simulink model "nichtlinearesModell_Kalman"  (R2016b)
settings: Solver=VariableStepAuto  StartTime=0.0  StopTime=30  RelTol=1e-3
values from neighbouring files (symbols this model uses):
  Ak = [A1                      E*C_s ... (first row only)    [StartSim.m]
  B1 = [0 b2 0 b4]'    [RiccatiBerechnung_Anlage.m]    (also in RiccatiBerechnunguPlot_Simulation.m; StartSim.m)
  Bk = [B1; zeros(1,size(B1,2))]    [StartSim.m]
  Ck = [C1 zeros(size(C1,1),1)]    [StartSim.m]
  K1 = 1    [RiccatiBerechnung_Anlage.m]    (also in RiccatiBerechnunguPlot_Simulation.m; StartSim.m)
  K2 = 1    [RiccatiBerechnung_Anlage.m]    (also in RiccatiBerechnunguPlot_Simulation.m; StartSim.m)
  Kk = P * Ck' / R    [StartSim.m]
  L_0 = 0.5    [RiccatiBerechnunguPlot_Simulation.m]    (also in StartSim.m)
  phi_0 = 0    [RiccatiBerechnunguPlot_Simulation.m]    (also in StartSim.m)
  r1 = 0.0191    [LQG.m]    (also in RiccatiBerechnung_Anlage.m = 0.046; RiccatiBerechnunguPlot_Simulation.m = 0.046; StartSim.m = 0.046)
  r2 = 0.015915    [LQG.m]    (also in RiccatiBerechnung_Anlage.m = 0.021975; RiccatiBerechnunguPlot_Simulation.m = 0.021975; StartSim.m = 0.025)
  T1 = 0.1    [LQG.m]    (also in RiccatiBerechnung_Anlage.m = 0.03032; RiccatiBerechnunguPlot_Simulation.m = 0.03032; StartSim.m = 0.03032)
  T2 = 0.1    [LQG.m]    (also in RiccatiBerechnung_Anlage.m = 0.0247; RiccatiBerechnunguPlot_Simulation.m = 0.0247; StartSim.m = 0.03032)
  ue1 = 6    [RiccatiBerechnung_Anlage.m]    (also in RiccatiBerechnunguPlot_Simulation.m; StartSim.m)
  ue2 = 3    [RiccatiBerechnung_Anlage.m]    (also in RiccatiBerechnunguPlot_Simulation.m; StartSim.m)
  x_0 = 2.54    [RiccatiBerechnunguPlot_Simulation.m]    (also in StartSim.m = 1.3)
undefined symbols (not defined in the file or in its folder): K
libraries: simulink_extras x3, simulink x2
settings Model: Creator=Patrick  LastModifiedBy=Patrick

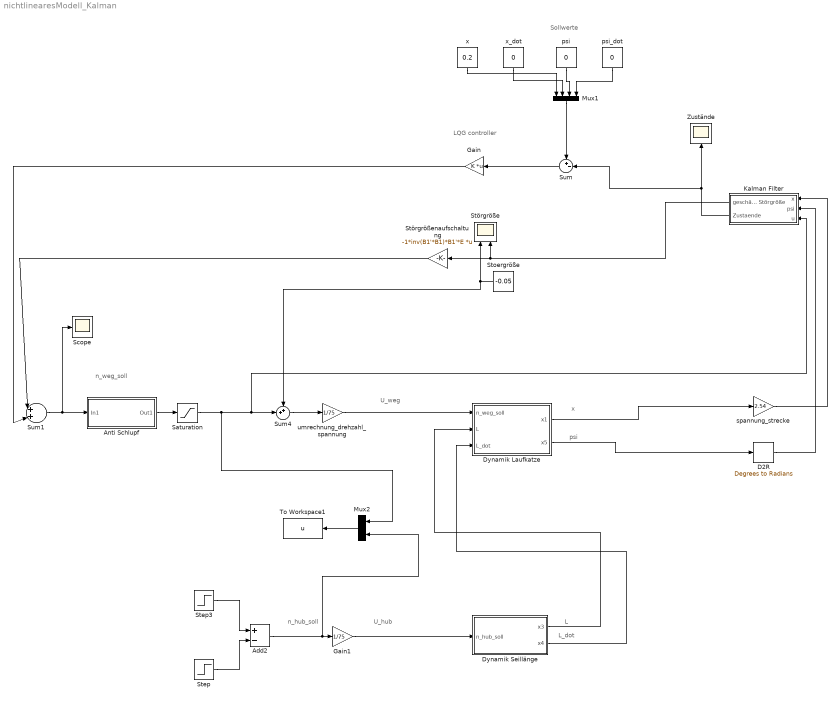
== system nichtlinearesModell_Kalman ==
  note: n_hub_soll
  note: U_hub
  note: L
  note: L_dot
  note: x
  note: psi
  note: LQG controller
  note: U_weg
  note: n_weg_soll
  note: Sollwerte
  Add2 : Sum  Inputs=+-
  Anti Schlupf : Subsystem
  D2R : simulink_extras/Transformations/Degrees to Radians
  Dynamik Laufkatze : Subsystem
  Dynamik Seillänge : Subsystem
  Gain : Gain  Gain=K  Multiplication=Matrix(K*u)
  Gain1 : Gain  Gain=1/75
  Kalman Filter : Subsystem
  Mux1 : Mux
  Mux2 : Mux  Inputs=2
  Saturation : Saturate  UpperLimit=75  LowerLimit=-75
  Scope : Scope
  Step : Step  Time=0  After=0  SampleTime=0
  Step3 : Step  Time=0  After=0  SampleTime=0
  Stoergröße : Constant  Value=-0.05
  Störgröße : Scope  NumInputPorts=2
  Störgrößenaufschaltung : Gain  Gain=-1*inv(B1'*B1)*B1'*E  Multiplication=Matrix(K*u)
  Sum : Sum  Inputs=+-|
  Sum1 : Sum  Inputs=|++|
  Sum4 : Sum  Inputs=++|
  To Workspace1 : ToWorkspace  VariableName=u  SampleTime=-1
  Zustände : Scope
  psi : Constant  Value=0
  psi_dot : Constant  Value=0
  spannung_strecke : Gain  Gain=2.54
  umrechnung_drehzahl_spannung : Gain  Gain=1/75
  x : Constant  Value=0.2
  x_dot : Constant  Value=0
  wires:
  Add2/1 -> Mux2/2, Gain1/1
  Gain1/1 -> Dynamik Seillänge/1(n_hub_soll)
  Step3/1 -> Add2/1
  Dynamik Seillänge/1(x3) -> Dynamik Laufkatze/2(L)
  Step/1 -> Add2/2
  Dynamik Seillänge/2(x4) -> Dynamik Laufkatze/3(L_dot)
  Mux2/1 -> To Workspace1/1
  Sum/1 -> Gain/1
  Gain/1 -> Sum1/2
  Dynamik Laufkatze/1(x1) -> spannung_strecke/1
  Kalman Filter/2(Zustaende) -> Zustände/1, Sum/2
  Stoergröße/1 -> Sum4/1, Störgröße/1
  umrechnung_drehzahl_spannung/1 -> Dynamik Laufkatze/1(n_weg_soll)
  Anti Schlupf/1(Out1) -> Saturation/1
  Kalman Filter/1(geschätzte Störgröße) -> Störgröße/2, Störgrößenaufschaltung/1
  Sum1/1 -> Scope/1, Anti Schlupf/1(In1)
  Saturation/1 -> Mux2/1, Kalman Filter/3(u), Sum4/2
  Mux1/1 -> Sum/1
  psi_dot/1 -> Mux1/4
  x_dot/1 -> Mux1/2
  psi/1 -> Mux1/3
  x/1 -> Mux1/1
  Sum4/1 -> umrechnung_drehzahl_spannung/1
  Störgrößenaufschaltung/1 -> Sum1/1
  Dynamik Laufkatze/2(x5) -> D2R/1
  spannung_strecke/1 -> Kalman Filter/1(x)
  D2R/1 -> Kalman Filter/2(psi)

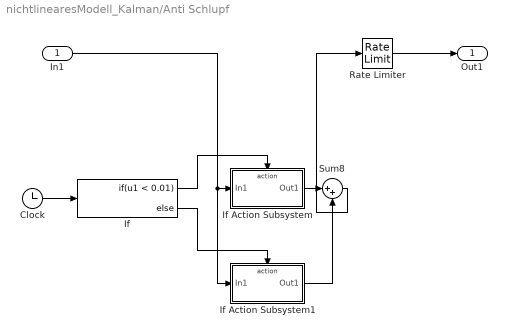
== system nichtlinearesModell_Kalman/Anti Schlupf ==
  In1 : Inport
  Clock : Clock
  If : If  IfExpression=u1 < 0.01
  If Action Subsystem : Subsystem  TreatAsAtomicUnit=on
  If Action Subsystem1 : Subsystem  TreatAsAtomicUnit=on
  Rate Limiter : RateLimiter  RisingSlewLimit=9.57  FallingSlewLimit=-9.57  SampleTimeMode=inherited
  Sum8 : Sum  Inputs=|++
  Out1 : Outport
  wires:
  In1/1 -> If Action Subsystem1/1(In1), If Action Subsystem/1(In1)
  If Action Subsystem/1(Out1) -> Sum8/1
  If Action Subsystem1/1(Out1) -> Sum8/2
  Sum8/1 -> Rate Limiter/1
  If/1 -> If Action Subsystem/Action
  If/2 -> If Action Subsystem1/Action
  Rate Limiter/1 -> Out1/1
  Clock/1 -> If/1

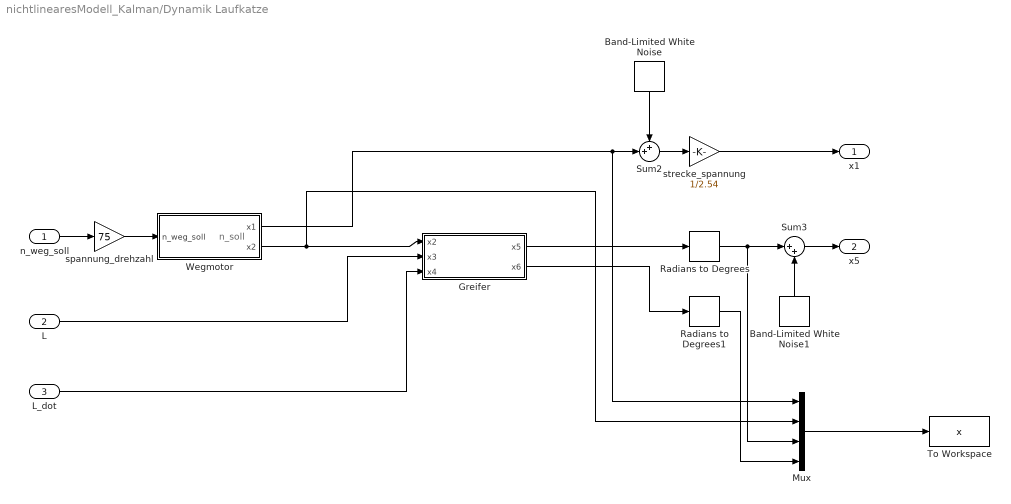
== system nichtlinearesModell_Kalman/Dynamik Laufkatze ==
  note: n_soll
  n_weg_soll : Inport
  L : Inport  Port=2
  L_dot : Inport  Port=3
  Band-Limited White Noise : simulink/Sources/Band-Limited White Noise  Cov=0.00000001  Ts=0.001  seed=[23341]
  Band-Limited White Noise1 : simulink/Sources/Band-Limited White Noise  Cov=0.00000001  Ts=0.001  seed=[23341]
  Greifer : Subsystem
  Mux : Mux
  Radians to Degrees : simulink_extras/Transformations/Radians to Degrees
  Radians to Degrees1 : simulink_extras/Transformations/Radians to Degrees
  Sum2 : Sum  Inputs=++|
  Sum3 : Sum  Inputs=|++
  To Workspace : ToWorkspace  VariableName=x  SampleTime=-1
  Wegmotor : Subsystem
  spannung_drehzahl : Gain  Gain=75
  strecke_spannung : Gain  Gain=1/2.54
  x1 : Outport
  x5 : Outport  Port=2
  wires:
  n_weg_soll/1 -> spannung_drehzahl/1
  Wegmotor/1(x1) -> Sum2/2, Mux/1
  Wegmotor/2(x2) -> Mux/2, Greifer/1(x2)
  Greifer/1(x5) -> Radians to Degrees/1
  Greifer/2(x6) -> Radians to Degrees1/1
  L/1 -> Greifer/2(x3)
  L_dot/1 -> Greifer/3(x4)
  spannung_drehzahl/1 -> Wegmotor/1(n_weg_soll)
  Radians to Degrees1/1 -> Mux/4
  Mux/1 -> To Workspace/1
  Radians to Degrees/1 -> Sum3/1, Mux/3
  strecke_spannung/1 -> x1/1
  Band-Limited White Noise1/1 -> Sum3/2
  Sum3/1 -> x5/1
  Sum2/1 -> strecke_spannung/1
  Band-Limited White Noise/1 -> Sum2/1

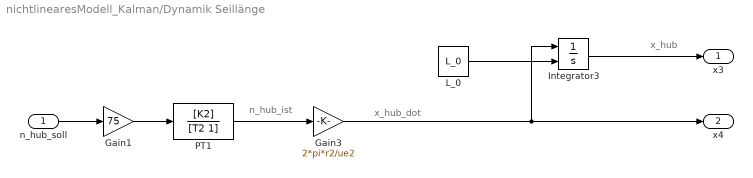
== system nichtlinearesModell_Kalman/Dynamik Seillänge ==
  note: n_hub_ist
  note: x_hub_dot
  note: x_hub
  n_hub_soll : Inport
  Gain1 : Gain  Gain=75
  Gain3 : Gain  Gain=2*pi*r2/ue2
  Integrator3 : Integrator  InitialConditionSource=external
  L_0 : Constant  Value=L_0
  PT1 : TransferFcn  Numerator=[K2]  Denominator=[T2 1]
  x3 : Outport
  x4 : Outport  Port=2
  wires:
  n_hub_soll/1 -> Gain1/1
  PT1/1 -> Gain3/1
  Integrator3/1 -> x3/1
  L_0/1 -> Integrator3/2
  Gain3/1 -> Integrator3/1, x4/1
  Gain1/1 -> PT1/1

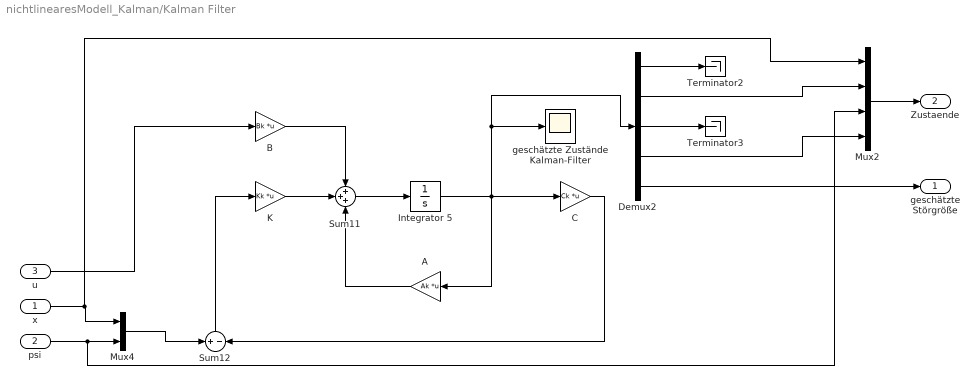
== system nichtlinearesModell_Kalman/Kalman Filter ==
  x : Inport
  psi : Inport  Port=2
  u : Inport  Port=3
  A : Gain  Gain=Ak  Multiplication=Matrix(K*u)
  B : Gain  Gain=Bk  Multiplication=Matrix(K*u)
  C : Gain  Gain=Ck  Multiplication=Matrix(K*u)
  Demux2 : Demux  Outputs=5
  Integrator 5 : Integrator
  K : Gain  Gain=Kk  Multiplication=Matrix(K*u)
  Mux2 : Mux
  Mux4 : Mux  Inputs=2
  Sum11 : Sum  Inputs=+++
  Sum12 : Sum  Inputs=+|-
  Terminator2 : Terminator
  Terminator3 : Terminator
  geschätzte Zustände Kalman-Filter : Scope
  geschätzte Störgröße : Outport
  Zustaende : Outport  Port=2
  wires:
  Integrator 5/1 -> geschätzte Zustände Kalman-Filter/1, Demux2/1, A/1, C/1
  Sum11/1 -> Integrator 5/1
  K/1 -> Sum11/2
  A/1 -> Sum11/3
  B/1 -> Sum11/1
  Sum12/1 -> K/1
  C/1 -> Sum12/2
  Mux4/1 -> Sum12/1
  Demux2/5 -> geschätzte Störgröße/1
  Demux2/1 -> Terminator2/1
  Demux2/3 -> Terminator3/1
  Demux2/2 -> Mux2/2
  Demux2/4 -> Mux2/4
  u/1 -> B/1
  x/1 -> Mux2/1, Mux4/1
  psi/1 -> Mux2/3, Mux4/2
  Mux2/1 -> Zustaende/1

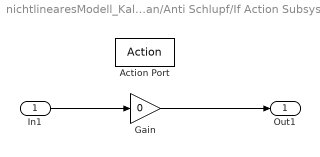
== system nichtlinearesModell_Kalman/Anti Schlupf/If Action Subsystem ==
  In1 : Inport
  Action Port : ActionPort  ActionType=then
  Gain : Gain  Gain=0
  Out1 : Outport
  wires:
  In1/1 -> Gain/1
  Gain/1 -> Out1/1

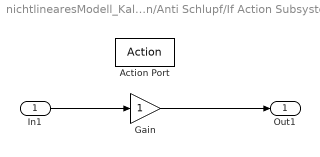
== system nichtlinearesModell_Kalman/Anti Schlupf/If Action Subsystem1 ==
  In1 : Inport
  Action Port : ActionPort  ActionType=else
  Gain : Gain
  Out1 : Outport
  wires:
  In1/1 -> Gain/1
  Gain/1 -> Out1/1

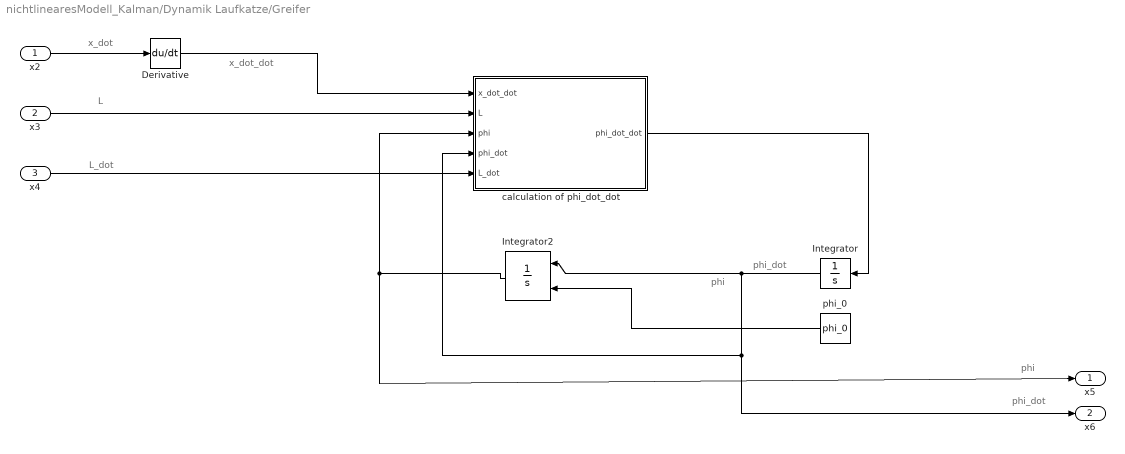
== system nichtlinearesModell_Kalman/Dynamik Laufkatze/Greifer ==
  note: phi
  note: phi
  note: x_dot
  note: L
  note: phi_dot
  note: phi_dot
  note: x_dot_dot
  note: L_dot
  x2 : Inport
  x3 : Inport  Port=2
  x4 : Inport  Port=3
  Derivative : Derivative
  Integrator : Integrator
  Integrator2 : Integrator  InitialConditionSource=external
  calculation of phi_dot_dot : MATLAB Function  TreatAsAtomicUnit=on
  phi_0 : Constant  Value=phi_0
  x5 : Outport
  x6 : Outport  Port=2
  wires:
  Derivative/1 -> calculation of phi_dot_dot/1(x_dot_dot)
  x2/1 -> Derivative/1
  Integrator/1 -> x6/1, calculation of phi_dot_dot/4(phi_dot), Integrator2/1
  x3/1 -> calculation of phi_dot_dot/2(L)
  calculation of phi_dot_dot/1(phi_dot_dot) -> Integrator/1
  Integrator2/1 -> x5/1, calculation of phi_dot_dot/3(phi)
  x4/1 -> calculation of phi_dot_dot/5(L_dot)
  phi_0/1 -> Integrator2/2

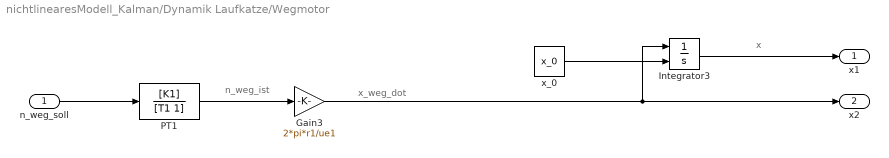
== system nichtlinearesModell_Kalman/Dynamik Laufkatze/Wegmotor ==
  note: n_weg_ist
  note: x
  note: x_weg_dot
  n_weg_soll : Inport
  Gain3 : Gain  Gain=2*pi*r1/ue1
  Integrator3 : Integrator  InitialConditionSource=external
  PT1 : TransferFcn  Numerator=[K1]  Denominator=[T1 1]
  x_0 : Constant  Value=x_0
  x1 : Outport
  x2 : Outport  Port=2
  wires:
  x_0/1 -> Integrator3/2
  n_weg_soll/1 -> PT1/1
  PT1/1 -> Gain3/1
  Integrator3/1 -> x1/1
  Gain3/1 -> Integrator3/1, x2/1

== matlab function nichtlinearesModell_Kalman/Dynamik Laufkatze/Greifer/calculation of phi_dot_dot ==
  data: x_dot_dot input; phi_dot_dot output; L input; phi input; phi_dot input; L_dot input
function phi_dot_dot = fcn(x_dot_dot,L,phi,phi_dot,L_dot)

phi_dot_dot = -(cos(phi)/L)*x_dot_dot-9.81/L*sin(phi)-2*L_dot*phi_dot;
